simulink model "part5"  (R2014a)
settings: Solver=ode45  StartTime=0.0  StopTime=10.0  RelTol=1e-3
settings Model: Creator=SuperUser  LastModifiedBy=SuperUser

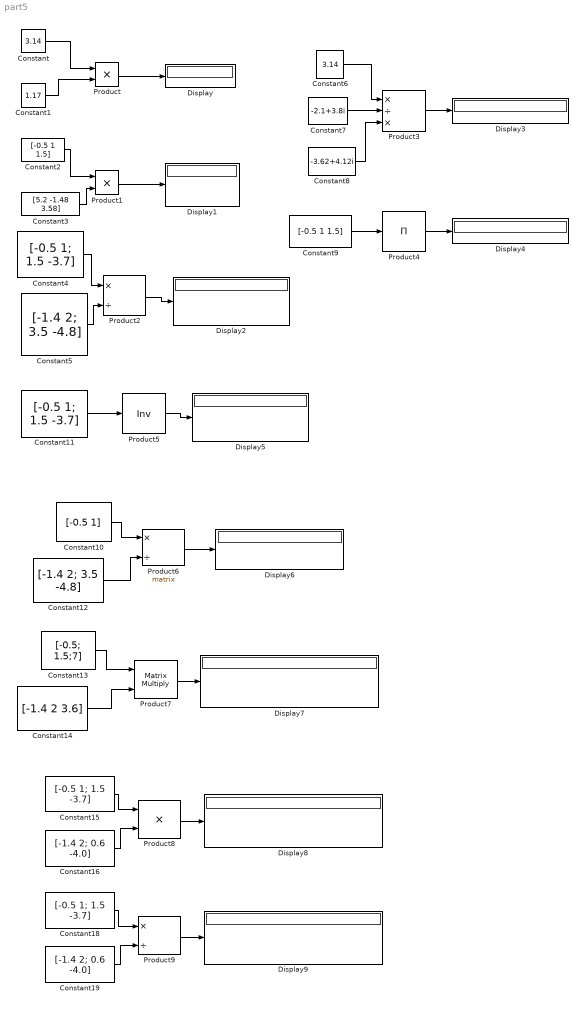
== system part5 ==
  Constant : Constant  Value=3.14
  Constant1 : Constant  Value=1.17
  Constant10 : Constant  Value=[-0.5 1]  VectorParams1D=off
  Constant11 : Constant  Value=[-0.5 1; 1.5 -3.7]
  Constant12 : Constant  Value=[-1.4 2; 3.5 -4.8]  VectorParams1D=off
  Constant13 : Constant  Value=[-0.5; 1.5;7]  VectorParams1D=off
  Constant14 : Constant  Value=[-1.4 2 3.6]  VectorParams1D=off
  Constant15 : Constant  Value=[-0.5 1; 1.5 -3.7]  VectorParams1D=off
  Constant16 : Constant  Value=[-1.4 2; 0.6 -4.0]  VectorParams1D=off
  Constant18 : Constant  Value=[-0.5 1; 1.5 -3.7]  VectorParams1D=off
  Constant19 : Constant  Value=[-1.4 2; 0.6 -4.0]  VectorParams1D=off
  Constant2 : Constant  Value=[-0.5 1 1.5]
  Constant3 : Constant  Value=[5.2 -1.48 3.58]
  Constant4 : Constant  Value=[-0.5 1; 1.5 -3.7]
  Constant5 : Constant  Value=[-1.4 2; 3.5 -4.8]
  Constant6 : Constant  Value=3.14
  Constant7 : Constant  Value=-2.1+3.8i
  Constant8 : Constant  Value=-3.62+4.12i
  Constant9 : Constant  Value=[-0.5 1 1.5]
  Display{,1..9} (10 alike) : Display
  Product : Product
  Product1 : Product
  Product2 : Product  Inputs=*/
  Product3 : Product  Inputs=*/*
  Product4 : Product  Inputs=1
  Product5 : Product  Inputs=/  Multiplication=Matrix(*)
  Product6 : Product  Inputs=*/  Multiplication=Matrix(*)
  Product7 : Product  Inputs=**  Multiplication=Matrix(*)
  Product8 : Product  Inputs=**
  Product9 : Product  Inputs=*/
  wires:
  Constant/1 -> Product/1
  Constant1/1 -> Product/2
  Product/1 -> Display/1
  Constant2/1 -> Product1/1
  Constant3/1 -> Product1/2
  Product1/1 -> Display1/1
  Constant4/1 -> Product2/1
  Constant5/1 -> Product2/2
  Product2/1 -> Display2/1
  Constant6/1 -> Product3/1
  Constant7/1 -> Product3/2
  Product3/1 -> Display3/1
  Constant8/1 -> Product3/3
  Constant9/1 -> Product4/1
  Product4/1 -> Display4/1
  Product5/1 -> Display5/1
  Constant11/1 -> Product5/1
  Constant10/1 -> Product6/1
  Constant12/1 -> Product6/2
  Product6/1 -> Display6/1
  Constant13/1 -> Product7/1
  Product7/1 -> Display7/1
  Constant14/1 -> Product7/2
  Constant15/1 -> Product8/1
  Product8/1 -> Display8/1
  Constant16/1 -> Product8/2
  Constant18/1 -> Product9/1
  Product9/1 -> Display9/1
  Constant19/1 -> Product9/2
